simulink model "Helicopter_Simulink_Model"  (R2015a)
settings: Solver=ode45  StartTime=0.0  StopTime=50  MaxStep=0.001  MinStep=0.0001  RelTol=1e-3
undefined symbols (not defined in the file): A, B, C, C_0, D, K_i, K_r, K_sf, L
settings Model: Creator=Owner  LastModifiedBy=Owner
settings HardwareCC: TargetLongLongMode=on  TargetIntDivRoundTo=Zero  TargetEndianess=LittleEndian  TargetHWDeviceType=MATLAB Host  ProdEqTarget=off
settings RTWCC: SystemTargetFile=rsim.tlc  TemplateMakefile=rsim_default_tmf  Description=Rapid Simulation Target
settings RSimTargetCC: ERTMultiwordTypeDef=System defined  ERTMultiwordLength=256

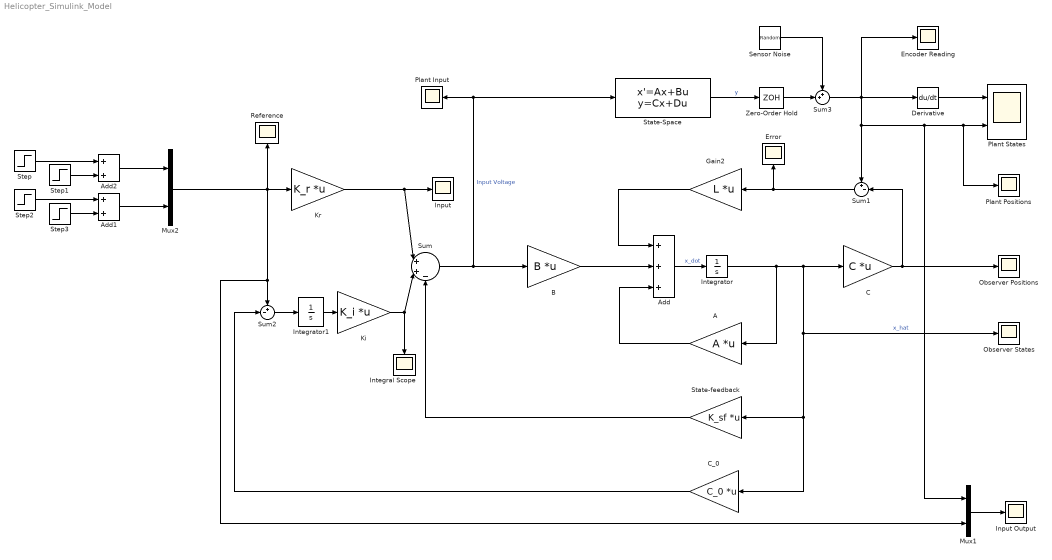
== system Helicopter_Simulink_Model ==
  A : Gain  Gain=A  Multiplication=Matrix(K*u)
  Add : Sum  Inputs=+++
  Add1 : Sum
  Add2 : Sum
  B : Gain  Gain=B  Multiplication=Matrix(K*u)
  C : Gain  Gain=C  Multiplication=Matrix(K*u)
  C_0 : Gain  Gain=C_0  Multiplication=Matrix(K*u)
  Derivative : Derivative
  Encoder Reading : Scope
      settings: SaveName=ScopeData6
  Error : Scope
      settings: SaveName=ScopeData3
  Gain2 : Gain  Gain=L  Multiplication=Matrix(K*u)
  Input : Scope
  Input Output : Scope
      settings: SaveName=io
  Integral Scope : Scope
      settings: SaveName=ScopeData11
  Integrator : Integrator
  Integrator1 : Integrator  LimitOutput=on  UpperSaturationLimit=0.7  LowerSaturationLimit=-0.7
  Ki : Gain  Gain=K_i  Multiplication=Matrix(K*u)
  Kr : Gain  Gain=K_r  Multiplication=Matrix(K*u)
  Mux1 : Mux  Inputs=2
  Mux2 : Mux  Inputs=2
  Observer Positions : Scope
      settings: SaveName=ScopeData4
  Observer States : Scope
      settings: SaveName=ScopeData2
  Plant Input : Scope
      settings: SaveName=ScopeData9
  Plant Positions : Scope
      settings: SaveName=ScopeData5
  Plant States : Scope  NumInputPorts=2
      settings: YMin=-5~-5  YMax=5~5
  Reference : Scope
      settings: SaveName=ScopeData8
  Sensor Noise : UniformRandomNumber  Minimum=-0.0002  Maximum=0.0002  SampleTime=0.012
  State-Space : StateSpace  A=A  B=B  C=C  D=D  X0=0
  State-feedback : Gain  Gain=K_sf  Multiplication=Matrix(K*u)
  Step : Step  Time=10  After=0.3  SampleTime=0
  Step1 : Step  Time=30  After=-0.3  SampleTime=0
  Step2 : Step  Time=10  After=0.8  SampleTime=0
  Step3 : Step  Time=30  After=-0.8  SampleTime=0
  Sum : Sum  Inputs=|++-
  Sum1 : Sum  Inputs=+-|
  Sum2 : Sum  Inputs=+-|
  Sum3 : Sum  Inputs=++|
  Zero-Order Hold : ZeroOrderHold  SampleTime=0.012
  wires:
  Sum/1 -> State-Space/1, Plant Input/1, B/1  "Input Voltage"
  B/1 -> Add/2
  A/1 -> Add/3
  Add/1 -> Integrator/1  "x_dot"
  Integrator/1 -> C/1, Observer States/1, C_0/1, State-feedback/1, A/1  "x_hat"
  Sum3/1 -> Encoder Reading/1, Derivative/1, Sum1/1, Mux1/1, Plant Positions/1, Plant States/2
  Gain2/1 -> Add/1
  Derivative/1 -> Plant States/1
  State-feedback/1 -> Sum/3
  Mux2/1 -> Reference/1, Kr/1, Mux1/2, Sum2/1
  Kr/1 -> Sum/1, Input/1
  Sum2/1 -> Integrator1/1
  C_0/1 -> Sum2/2
  Ki/1 -> Sum/2, Integral Scope/1
  Integrator1/1 -> Ki/1
  Sum1/1 -> Error/1, Gain2/1
  Sensor Noise/1 -> Sum3/1
  State-Space/1 -> Zero-Order Hold/1  "y"
  Zero-Order Hold/1 -> Sum3/2
  Mux1/1 -> Input Output/1
  C/1 -> Observer Positions/1, Sum1/2
  Add1/1 -> Mux2/2
  Add2/1 -> Mux2/1
  Step/1 -> Add2/1
  Step1/1 -> Add2/2
  Step2/1 -> Add1/1
  Step3/1 -> Add1/2
